simulink model "top_level"  (R2018b)
settings: Solver=VariableStepAuto  StartTime=0.0  StopTime=10.0  RelTol=1e-3
undefined symbols (not defined in the file or in its folder): sub
settings Model: Creator=Danijel  LastModifiedBy=Danijel

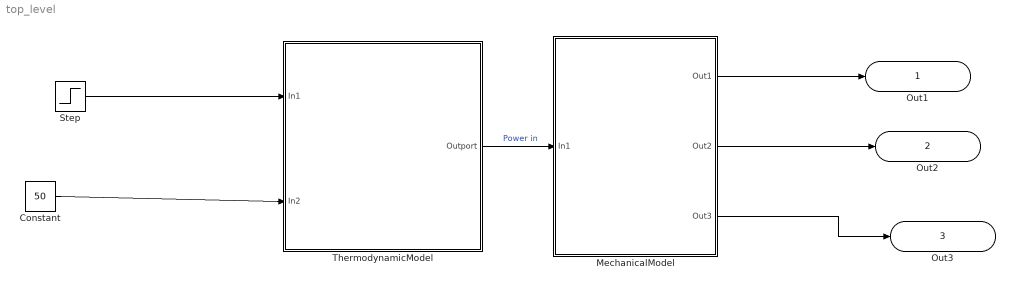
== system top_level ==
  Constant : Constant  Value=50
  MechanicalModel : Subsystem
  Step : Step  Time=5  Before=0.9  After=0.8  SampleTime=0
  ThermodynamicModel : Subsystem
  Out1 : Outport
  Out2 : Outport  Port=2
  Out3 : Outport  Port=3
  wires:
  Step/1 -> ThermodynamicModel/1(In1)
  Constant/1 -> ThermodynamicModel/2(In2)
  ThermodynamicModel/1(Outport) -> MechanicalModel/1(In1)  "Power in"
  MechanicalModel/1(Out1) -> Out1/1
  MechanicalModel/2(Out2) -> Out2/1
  MechanicalModel/3(Out3) -> Out3/1

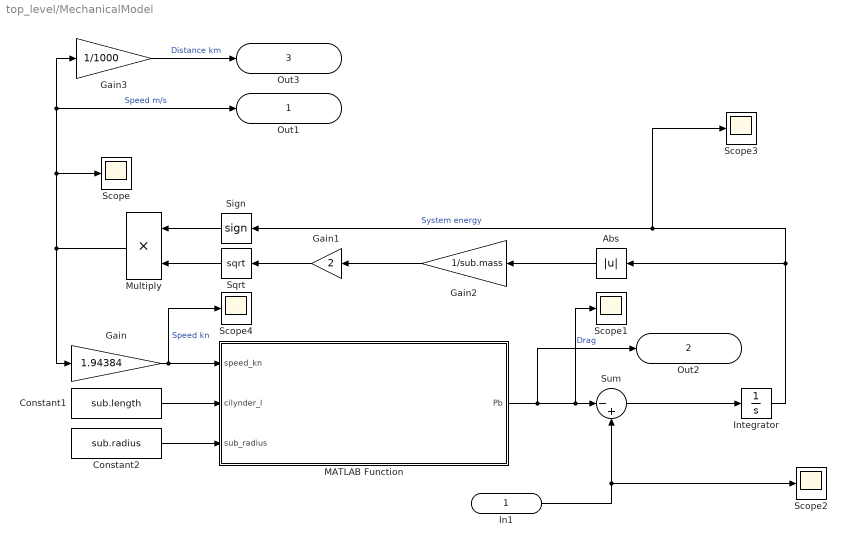
== system top_level/MechanicalModel ==
  In1 : Inport
  Abs : Abs
  Constant1 : Constant  Value=sub.length
  Constant2 : Constant  Value=sub.radius
  Gain : Gain  Gain=1.94384
  Gain1 : Gain  Gain=2
  Gain2 : Gain  Gain=1/sub.mass
  Gain3 : Gain  Gain=1/1000
  Integrator : Integrator
  MATLAB Function : MATLAB Function  TreatAsAtomicUnit=on
  Multiply : Product
  Scope{,1..4} (5 alike) : Scope
  Sign : Signum
  Sqrt : Sqrt  SaturateOnIntegerOverflow=on
  Sum : Sum  Inputs=|-+
  Out1 : Outport
  Out2 : Outport  Port=2
  Out3 : Outport  Port=3
  wires:
  Constant1/1 -> MATLAB Function/2(cilynder_l)
  Integrator/1 -> Scope3/1, Sign/1, Abs/1  "System energy"
  Gain3/1 -> Out3/1  "Distance km"
  In1/1 -> Sum/2, Scope2/1
  Sign/1 -> Multiply/1
  MATLAB Function/1(Pb) -> Out2/1, Sum/1, Scope1/1  "Drag"
  Abs/1 -> Gain2/1
  Multiply/1 -> Gain/1, Out1/1, Gain3/1, Scope/1  "Speed m/s"
  Sqrt/1 -> Multiply/2
  Sum/1 -> Integrator/1
  Gain2/1 -> Gain1/1
  Gain/1 -> Scope4/1, MATLAB Function/1(speed_kn)  "Speed kn"
  Gain1/1 -> Sqrt/1
  Constant2/1 -> MATLAB Function/3(sub_radius)

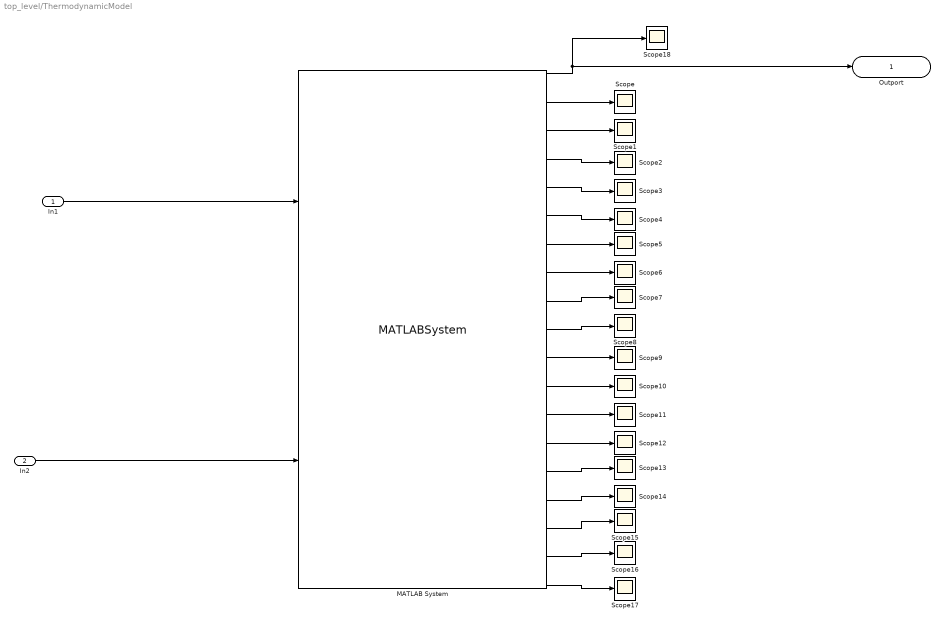
== system top_level/ThermodynamicModel ==
  In1 : Inport
  In2 : Inport  Port=2
  MATLAB System : MATLABSystem  System=PowerGenerationS  InitMass=5000  TurbID=18  PipeID=1  PipeL=3.29  EvapPipeNR=280  SuperPipeNr=63  EvapFGfrac=0.949643535090430  ComprID=23  N1=0.91  L1=0.41  N2=1  L2=0.6  TretInit=210  FuelPumpID=13  SimulateUsing=Interpreted execution
      mask Type: PowerGenerationS
      mask Display:
      | disp('PowerGenerationS');
      | port_label('input',1,'pumpSpeed');
      | port_label('input',2,'depth');
      | port_label('output',1,'Power');
      | port_label('output',2,'fuelFlow_kgs');
      | port_label('output',3,'fuel_kg');
      | port_label('output',4,'Tcomb');
      | port_label('output',5,'TevapOut');
      | port_label('output',6,'TsuperOut');
      | port_label('output',7,'Tret');
      | port_label('output',8,'qmSteam_kg_s');
      | port_label('output',9,'pThr_bar');
      | port_label('output',10,'TsteamTurb');
      | port_label('output',11,'vapFrac');
      | port_label('output',12,'eta_turb');
      | port_label('output',13,'evapSpeed');
      | port_label('output',14,'superSpeed');
      | port_label('output',15,'evapAlfaFG');
      | port_label('output',16,'superAlfaFG');
      | port_label('output',17,'evapHTC');
      | port_label('output',18,'superHTC');
      | port_label('output',19,'system_efficiency');
  Scope{,1..18} (19 alike) : Scope
  Outport : Outport
  wires:
  MATLAB System/8 -> Scope6/1
  MATLAB System/9 -> Scope7/1
  MATLAB System/10 -> Scope8/1
  MATLAB System/19 -> Scope17/1
  MATLAB System/16 -> Scope14/1
  MATLAB System/7 -> Scope5/1
  MATLAB System/14 -> Scope12/1
  MATLAB System/1 -> Outport/1, Scope18/1
  MATLAB System/17 -> Scope15/1
  MATLAB System/18 -> Scope16/1
  MATLAB System/11 -> Scope9/1
  MATLAB System/2 -> Scope/1
  MATLAB System/15 -> Scope13/1
  In2/1 -> MATLAB System/2
  MATLAB System/13 -> Scope11/1
  MATLAB System/4 -> Scope2/1
  MATLAB System/3 -> Scope1/1
  MATLAB System/5 -> Scope3/1
  MATLAB System/12 -> Scope10/1
  MATLAB System/6 -> Scope4/1
  In1/1 -> MATLAB System/1

== matlab function top_level/MechanicalModel/MATLAB Function ==
  data: speed_kn input; Pb output; cilynder_l input; sub_radius input
function Pb  = sub_power(speed_kn,cilynder_l, sub_radius)
%sub_power Summary of this function goes here
%   Detailed explanation goes here



% Densities
row = 1025; % kg/m^3 - Salt water
roc = 7850; % kg/m^3 - Steel
rop = 1300; % kg/m^3 - Plastics

% Physical constants
g = 9.81; % m/s^2

negative = 1;

if speed_kn < 0
    negative = -1;
    speed_kn = speed_kn * -1;
end

% Surface

sub_length = cilynder_l + 2 * sub_radius;

sur_cylinder = 2 * sub_radius * pi * cilynder_l;
sur_sphere =  4 * sub_radius^2 * pi;

sub_surface = sur_cylinder + sur_sphere;

% Volume

vol_cylinder = sub_radius^2 * cilynder_l * pi; % m^3
vol_sphere = 4/3 * sub_radius^3 * pi; % m^3
sub_volume = vol_cylinder + vol_sphere; % m^3

istisnina = row * sub_volume; % t

CB =  sub_volume / (sub_length * 2 * sub_radius * 2 * sub_radius); % Block coefficient





speed_ms = speed_kn * 0.514444;

ni = 0.000001187; % m^2/s - Kinematic vicscosity 
Rn = speed_ms * sub_length / ni; % Reynolds_number

CF = 0.075/(log10(Rn)-2)^2; % Friction coefficient

Fn = speed_ms /sqrt(9.08665 * sub_length);


k=-0.095+25.6 *CB/((sub_length/(2*sub_radius))^2);

CT = CF * (1 + k);

Re = CT * 0.5 * row * speed_ms^2 * sub_surface / 1000; % kW
Pe = Re * speed_ms; % kW
Pb1 = Pe/(0.5*0.98);
Pb = Pb1/0.85; % kW


Pb = Pb * negative;

end
